simulink model "cv_intersect_rectangles"  (Simulink 6.0)
settings: Solver=ode45  StartTime=0.0  StopTime=10.0  RelTol=1e-3
settings Model: RecordCoverage=on  CovMetricSettings=dcmtw  CovHTMLOptions=-aTS=1 -bRG=1 -bTC=0 -hTR=0 -nFC=0 -scm=1 -bcm=1  Creator=The MathWorks Inc.  LastModifiedBy=batserve  ExtModeAutoUpdateStatusClock=off  ProdHWDeviceType=Specified
settings DataIOCC: SignalLoggingName=logsOut
settings DebuggingCC: CheckExecutionContextPreStartOutputMsg=on  CheckExecutionContextRuntimeOutputMsg=on  SolverPrmCheckMsg=none
settings HardwareCC: ProdHWDeviceType=Specified

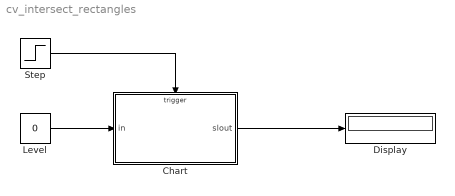
== system cv_intersect_rectangles ==
  Chart : Stateflow chart  PropExecContextAcrossSSBoundary=on
  Display : Display
  Level : Constant  Value=0
  Step : Step  SampleTime=0
  wires:
  Step/1 -> Chart/Trigger
  Chart/1(slout) -> Display/1
  Level/1 -> Chart/1(in)

== matlab function Chart ==
  data: rect1 function_input double size=4; rect2 function_input double size=4; out function_output double; out function_output double; level function_input double; slout output double; in input double
  events: event input RISING_EDGE_EVENT
function out = rct_intersect(rect1,rect2) 
% RECT_INTERSECT - Determine if two rectangles intersect
    
    left1 = rect1(1);
    bottom1 = rect1(2);
    right1 = left1 + rect1(3);
    top1 = bottom1 + rect1(4);
 
    left2 = rect2(1);
    bottom2 = rect2(2);
    right2 = left2 + rect2(3);
    top2 = bottom2 + rect2(4);
    
    out = 1;

    if (top1 < bottom2 || top2 < bottom1)
        out = 0;
    else
        if (right1 < left2 || right2 < left1)
            out = 0;
        end
    end

== matlab function Chart ==
function out = run(level)

% Calls to achieve statement coverage
out = intersect([0 1.25 1 1]',[0 0 1 1]', 1);
out = intersect([1.5 1.25 1 1]',[2.75 .75 1 1]', 2);

if level>0
    % Call to achieve decision coverage
    out = intersect([4.5 1.25 1 1]',[5 .75 1 1]', 3);
    
    if level>1
        % Call to achieve Condition and MCDC coverage
        out = intersect([6.5 0 1 1]',[6.5 1.25 1 1]', 4);
        out = intersect([9.25 1.25 1 1]',[8 .75 1 1]', 5);
    end
end

function out = intersect(rectOne, rectTwo, idx)
    display_intersect_rect(rectOne, 0, idx);
    display_intersect_rect(rectTwo, 2, idx);
    out = rct_intersect(rectOne, rectTwo);
